simulink model "ff18"  (R2015b)
settings: Solver=VariableStepAuto  StartTime=0.0  StopTime=10.0  RelTol=1e-3
undefined symbols (not defined in the file): a, b, c, Csfl, Csfr, Csrl, Csrr, d, Ksfl, Ksfr, Ksrl, Ksrr, M, S
settings Model: Creator=Guest  LastModifiedBy=Guest

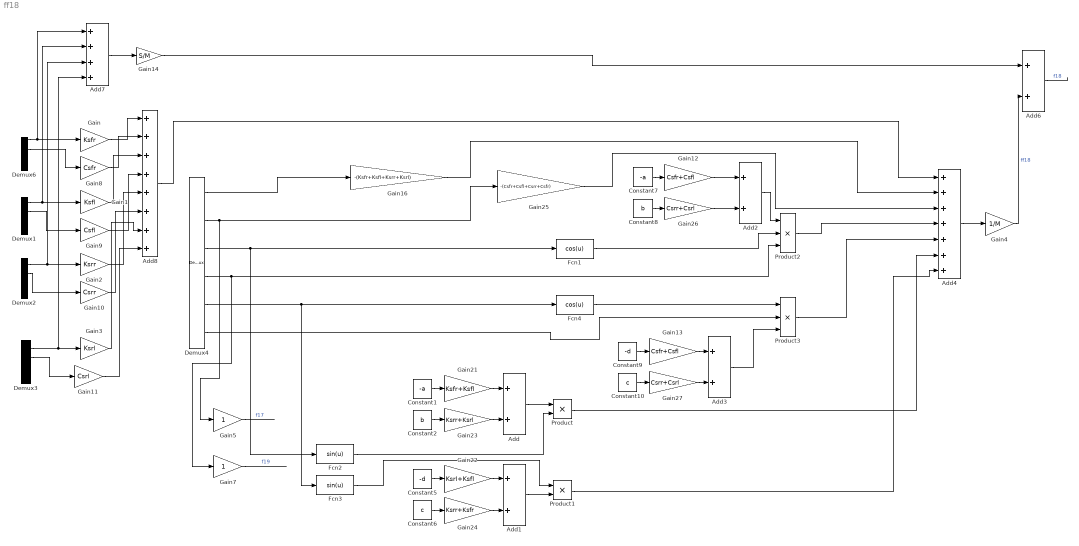
== system ff18 ==
  Add{,1..3,6} (5 alike) : Sum
  Add4 : Sum  Inputs=+++++++
  Add7 : Sum  Inputs=++++
  Add8 : Sum  Inputs=++++++++
  Constant1 : Constant  Value=-a
  Constant10 : Constant  Value=c
  Constant2 : Constant  Value=b
  Constant5 : Constant  Value=-d
  Constant6 : Constant  Value=c
  Constant7 : Constant  Value=-a
  Constant8 : Constant  Value=b
  Constant9 : Constant  Value=-d
  Demux{1..3,6} (4 alike) : Demux
  Demux4 : Demux  Outputs=6
  Fcn1 : Fcn  Expr=cos(u)
  Fcn2 : Fcn  Expr=sin(u)
  Fcn3 : Fcn  Expr=sin(u)
  Fcn4 : Fcn  Expr=cos(u)
  Gain : Gain  Gain=Ksfr
  Gain1 : Gain  Gain=Ksfl
  Gain10 : Gain  Gain=Csrr
  Gain11 : Gain  Gain=Csrl
  Gain12 : Gain  Gain=Csfr+Csfl
  Gain13 : Gain  Gain=Csfr+Csfl
  Gain14 : Gain  Gain=S/M
  Gain16 : Gain  Gain=-(Ksfr+Ksfl+Ksrr+Ksrl)
  Gain2 : Gain  Gain=Ksrr
  Gain21 : Gain  Gain=Ksfr+Ksfl
  Gain22 : Gain  Gain=Ksrl+Ksfl
  Gain23 : Gain  Gain=Ksrr+Ksrl
  Gain24 : Gain  Gain=Ksrr+Ksfr
  Gain25 : Gain  Gain=-(Csfr+Csfl+Csrr+Csfr)
  Gain26 : Gain  Gain=Csrr+Csrl
  Gain27 : Gain  Gain=Csrr+Csrl
  Gain3 : Gain  Gain=Ksrl
  Gain4 : Gain  Gain=1/M
  Gain5 : Gain
  Gain7 : Gain
  Gain8 : Gain  Gain=Csfr
  Gain9 : Gain  Gain=Csfl
  Product : Product
  Product1 : Product
  Product2 : Product  Inputs=3
  Product3 : Product  Inputs=3
  wires:
  Demux6/1 -> Add7/1, Gain/1
  Demux1/1 -> Gain1/1, Add7/2
  Demux2/1 -> Gain2/1, Add7/3
  Demux3/1 -> Add7/4, Gain3/1
  Demux4/1 -> Gain16/1
  Demux4/3 -> Fcn2/1, Fcn1/1
  Gain21/1 -> Add/1
  Constant1/1 -> Gain21/1
  Gain23/1 -> Add/2
  Constant2/1 -> Gain23/1
  Add/1 -> Product/1
  Fcn2/1 -> Product/2
  Demux4/5 -> Fcn3/1, Fcn4/1
  Gain22/1 -> Add1/1
  Gain24/1 -> Add1/2
  Constant5/1 -> Gain22/1
  Constant6/1 -> Gain24/1
  Add1/1 -> Product1/2
  Fcn3/1 -> Product1/1
  Demux4/2 -> Gain5/1, Gain25/1
  Demux4/4 -> Gain7/1, Product2/3
  Fcn1/1 -> Product2/2
  Gain12/1 -> Add2/1
  Constant7/1 -> Gain12/1
  Gain26/1 -> Add2/2
  Constant8/1 -> Gain26/1
  Add2/1 -> Product2/1
  Gain13/1 -> Add3/1
  Constant9/1 -> Gain13/1
  Gain27/1 -> Add3/2
  Constant10/1 -> Gain27/1
  Fcn4/1 -> Product3/1
  Demux4/6 -> Product3/2
  Add3/1 -> Product3/3
  Product/1 -> Add4/6
  Product1/1 -> Add4/7
  Add4/1 -> Gain4/1
  Gain14/1 -> Add6/1
  Gain4/1 -> Add6/2  "ff18"
  Add6/1 -> ?  "f18"
  Gain5/1 -> ?  "f17"
  Gain7/1 -> ?  "f19"
  Demux6/2 -> Gain8/1
  Demux1/2 -> Gain9/1
  Demux2/2 -> Gain10/1
  Demux3/2 -> Gain11/1
  Add7/1 -> Gain14/1
  Gain/1 -> Add8/1
  Gain8/1 -> Add8/2
  Gain1/1 -> Add8/3
  Gain9/1 -> Add8/4
  Gain2/1 -> Add8/5
  Gain10/1 -> Add8/6
  Gain3/1 -> Add8/7
  Gain11/1 -> Add8/8
  Product3/1 -> Add4/5
  Product2/1 -> Add4/4
  Gain25/1 -> Add4/3
  Gain16/1 -> Add4/2
  Add8/1 -> Add4/1
